simulink model "EV_drive"  (Simulink 8.7)
settings: Solver=VariableStepAuto  StartTime=0.0  StopTime=100  RelTol=1e-3
undefined symbols (not defined in the file): sigbuilder_block
settings Model: Creator=Gorkem  LastModifiedBy=Gorkem
settings DataIOCC: LimitDataPoints=off  SaveFormat=Dataset
settings DebuggingCC: UnderspecifiedInitializationDetection=Simplified  MergeDetectMultiDrivingBlocksExec=error
settings HardwareCC: ProdBitPerPointer=64  ProdLargestAtomicFloat=Float  ProdIntDivRoundTo=Zero  ProdEndianess=LittleEndian  ProdWordSize=64  ProdHWDeviceType=Intel->x86-64 (Windows64)
settings ModelReferenceCC: PropagateSignalLabelsOutOfModel=on
settings ConfigComp: CovModelRefEnable=off

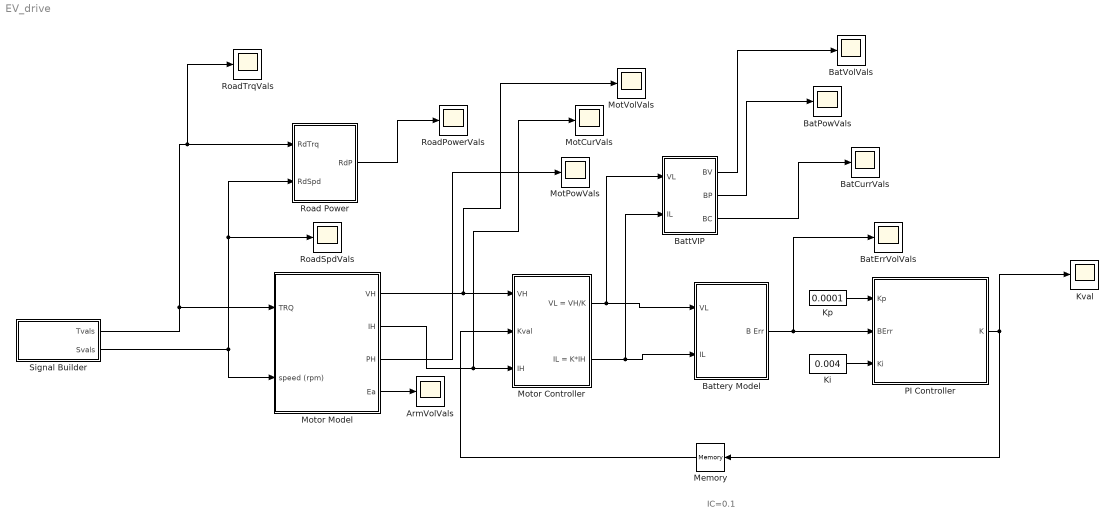
== system EV_drive ==
  note: IC=0.1
  ArmVolVals : Scope
  BatCurrVals : Scope
  BatErrVolVals : Scope
  BatPowVals : Scope
  BatVolVals : Scope
  BattVIP : Subsystem
  Battery Model : Subsystem
  Ki : Constant  Value=0.004
  Kp : Constant  Value=0.0001
  Kval : Scope
  Memory : Memory  X0=0.1
  MotCurVals : Scope
  MotPowVals : Scope
  MotVolVals : Scope
  Motor Controller : Subsystem
  Motor Model : Subsystem
  PI Controller : Subsystem
  Road Power : Subsystem
  RoadPowerVals : Scope
  RoadSpdVals : Scope
  RoadTrqVals : Scope
  Signal Builder : Subsystem  Tag=STV Subsys  LoadFcn=sigbuilder_block('load');  StartFcn=sigbuilder_block('start');  StopFcn=sigbuilder_block('stop');  ClipboardFcn=sigbuilder_block('clipboard');  mask(Sigbuilder block){}
      mask help: Simulink:masks:SigbuilderBlock_MD
      mask init:
      | if ~strcmp(get_param(bdroot(gcbh),'SimulationStatus'),'stopped') tuvar = sigbuilder_block('maskInit'); end
      settings: CopyFcn=sigbuilder_block('copy');  DeleteFcn=sigbuilder_block('delete');  ModelCloseFcn=sigbuilder_block('modelClose');  PreSaveFcn=sigbuilder_block('preSave');  PauseFcn=sigbuilder_block('pause');  ContinueFcn=sigbuilder_block('continue');  NameChangeFcn=sigbuilder_block('namechange');  OpenFcn=sigbuilder_block('open',[3 30 1018.5 447.75 ]);  CloseFcn=sigbuilder_block('close');
      mask Display: plot(0, 0, 100, 100,[2, 2, 32, 32, 2], [68, 8, 8, 68, 68],[32, 2], [38, 38], [32, 19, 2],[53, 60, 44], [32, 17, 17, 2],[16, 16, 31, 31]);txt = getActiveGroup(gcbh);text(2, 100, txt,'verticalAlignment', 'top');
  wires:
  Road Power/1(RdP) -> RoadPowerVals/1
  Motor Model/1(VH) -> MotVolVals/1, Motor Controller/1(VH)
  Motor Model/2(IH) -> MotCurVals/1, Motor Controller/3(IH)
  Motor Model/3(PH) -> MotPowVals/1
  Motor Controller/1(VL = VH/K) -> BattVIP/1(VL), Battery Model/1(VL)
  Motor Controller/2(IL = K*IH) -> BattVIP/2(IL), Battery Model/2(IL)
  BattVIP/1(BV) -> BatVolVals/1
  BattVIP/2(BP) -> BatPowVals/1
  BattVIP/3(BC) -> BatCurrVals/1
  Ki/1 -> PI Controller/3(Ki)
  Kp/1 -> PI Controller/1(Kp)
  Battery Model/1(B Err) -> BatErrVolVals/1, PI Controller/2(BErr)
  PI Controller/1(K) -> Memory/1, Kval/1
  Memory/1 -> Motor Controller/2(Kval)
  Signal Builder/1(Tvals) -> RoadTrqVals/1, Road Power/1(RdTrq), Motor Model/1(TRQ)
  Signal Builder/2(Svals) -> Motor Model/2(speed (rpm)), RoadSpdVals/1, Road Power/2(RdSpd)
  Motor Model/4(Ea) -> ArmVolVals/1

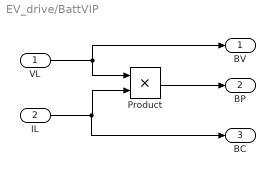
== system EV_drive/BattVIP ==
  VL : Inport
  IL : Inport  Port=2
  Product : Product
  BV : Outport
  BP : Outport  Port=2
  BC : Outport  Port=3
  wires:
  Product/1 -> BP/1
  VL/1 -> BV/1, Product/1
  IL/1 -> BC/1, Product/2

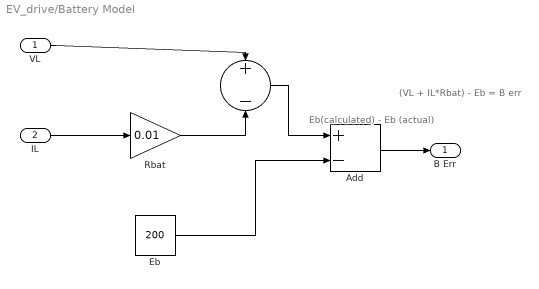
== system EV_drive/Battery Model ==
  note: (VL + IL*Rbat) - Eb = B err
  note: Eb(calculated) - Eb (actual)
  VL : Inport
  IL : Inport  Port=2
  "     " : Sum  Inputs=+-
  Add : Sum  Inputs=+-
  Eb : Constant  Value=200
  Rbat : Gain  Gain=0.01
  B Err : Outport
  wires:
  IL/1 -> Rbat/1
  Eb/1 -> Add/2
  Add/1 -> B Err/1
  Rbat/1 -> "     "/2
  "     "/1 -> Add/1
  VL/1 -> "     "/1

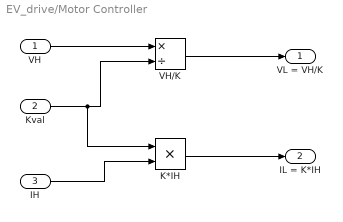
== system EV_drive/Motor Controller ==
  VH : Inport
  Kval : Inport  Port=2
  IH : Inport  Port=3
  K*IH : Product
  VH/K : Product  Inputs=*/
  VL = VH/K : Outport
  IL = K*IH : Outport  Port=2
  wires:
  IH/1 -> K*IH/2
  VH/1 -> VH/K/1
  K*IH/1 -> IL = K*IH/1
  VH/K/1 -> VL = VH/K/1
  Kval/1 -> VH/K/2, K*IH/1

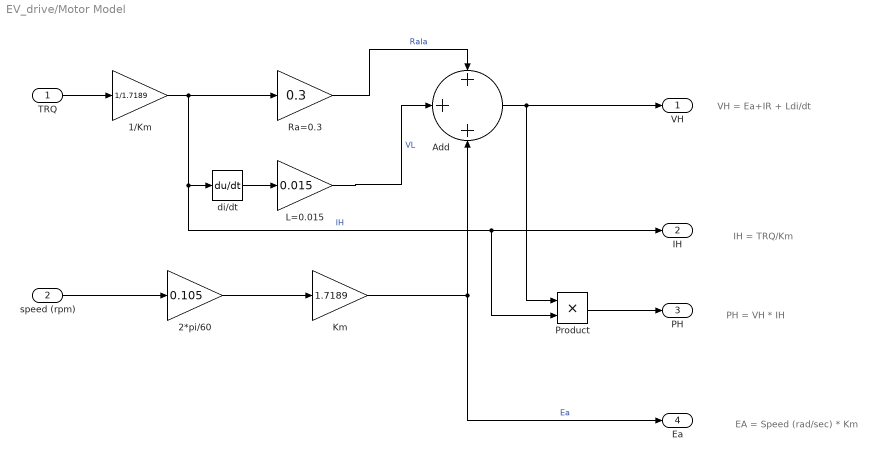
== system EV_drive/Motor Model ==
  note: EA = Speed (rad/sec) * Km
  note: PH = VH * IH
  note: IH = TRQ/Km
  note: VH = Ea+IR + Ldi/dt
  TRQ : Inport
  speed (rpm) : Inport  Port=2
  "            Add" : Sum  Inputs=+++  OutMin=[3]  OutMax=[19]
  1/Km : Gain  Gain=1/1.7189
  2*pi/60 : Gain  Gain=0.105
  Km : Gain  Gain=1.7189  OutMin=[1]  OutMax=[9]
  L=0.015 : Gain  Gain=0.015
  Product : Product
  "Ra=0.3 " : Gain  Gain=0.3
  di/dt : Derivative
  VH : Outport
  IH : Outport  Port=2
  PH : Outport  Port=3
  Ea : Outport  Port=4
  wires:
  TRQ/1 -> 1/Km/1
  speed (rpm)/1 -> 2*pi/60/1
  2*pi/60/1 -> Km/1
  di/dt/1 -> L=0.015/1
  "            Add"/1 -> VH/1, Product/1
  1/Km/1 -> IH/1, Product/2, di/dt/1, "Ra=0.3 "/1  "IH"
  L=0.015/1 -> "            Add"/2  "VL"
  Km/1 -> Ea/1, "            Add"/3  "Ea"
  Product/1 -> PH/1
  "Ra=0.3 "/1 -> "            Add"/1  "RaIa"

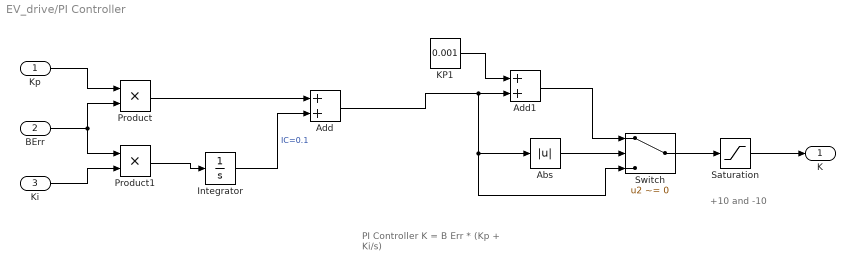
== system EV_drive/PI Controller ==
  note: PI Controller
      |
      | K = B Err * (Kp + Ki/s)
  note: +10 and -10
  Kp : Inport
  BErr : Inport  Port=2
  Ki : Inport  Port=3
  Abs : Abs
  Add : Sum
  Add1 : Sum
  Integrator : Integrator  InitialCondition=0.1  LimitOutput=on  IgnoreLimit=on
  KP1 : Constant  Value=0.001
  Product : Product
  Product1 : Product
  Saturation : Saturate  UpperLimit=+10  LowerLimit=-10
  Switch : Switch  Criteria=u2 ~= 0
  K : Outport
  wires:
  Kp/1 -> Product/1
  Abs/1 -> Switch/2
  Add/1 -> Switch/3, Abs/1, Add1/2
  BErr/1 -> Product1/1, Product/2
  Ki/1 -> Product1/2
  Product1/1 -> Integrator/1
  Switch/1 -> Saturation/1
  KP1/1 -> Add1/1
  Product/1 -> Add/1
  Saturation/1 -> K/1
  Integrator/1 -> Add/2  "IC=0.1"
  Add1/1 -> Switch/1

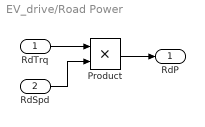
== system EV_drive/Road Power ==
  RdTrq : Inport
  RdSpd : Inport  Port=2
  Product : Product
  RdP : Outport
  wires:
  Product/1 -> RdP/1
  RdSpd/1 -> Product/2
  RdTrq/1 -> Product/1

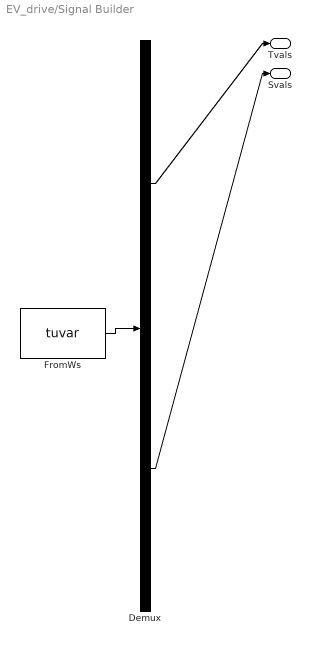
== system EV_drive/Signal Builder ==
  Demux : Demux  Tag=STV Demux  Outputs=2
  FromWs : FromWorkspace  Tag=STV FromWs  VariableName=tuvar  SampleTime=0  SigBuilderData=DataTag0  VnvData=DataTag1
      SigBuilderData=|
      | common.afterFinalStr = 'Extrapolate'
      | common.sampleTime = 0
      | dataSet.timeRange = [0 100]
      | dataSet.name = 'Group 1'
      | sbobj.Groups.Name = 'Group 1'
      | sbobj.Groups.Signals(1).Name = 'Tvals'
      | sbobj.Groups.Signals(1).XData = [0 5 10 15 50 55 80 85 100]
      | sbobj.Groups.Signals(1).YData = [0 330 330 160 160 -220 -220 0 0]
      | sbobj.Groups.Signals(2).Name = 'Svals'
      | sbobj.Groups.Signals(2).XData = [0 5 50 85 100]
      | sbobj.Groups.Signals(2).YData = [0 2000 3000 1000 1000]
      | sbobj.Groups.TimeRange = [0 100]
  Tvals : Outport  Tag=STV Outport
  Svals : Outport  Tag=STV Outport  Port=2
  wires:
  FromWs/1 -> Demux/1
  Demux/1 -> Tvals/1
  Demux/2 -> Svals/1
